simulink model "BraccioWithMotorsAndPIDandRL2020"  (R2020a)
settings: Solver=ode1be  StartTime=0.0  StopTime=14  FixedStep=0.01  RelTol=1e-3
values from neighbouring files (symbols this model uses):
  Z = [error; uold]    [RLNoLoop.m]
undefined symbols (not defined in the file or in its folder): X, Y
libraries: sm_lib x156, nesl_utility x52, simulink x12
(part 5 of 5)

== system BraccioWithMotorsAndPIDandRL2020/Subsystem3/link2 ==
  ReferenceFrame : sm_lib/Frames and Transforms/Reference Frame
  elbow_AxisTransform : sm_lib/Frames and Transforms/Rigid Transform  TranslationMethod=Cartesian  TranslationStandardOffset=0  TranslationStandardOffsetUnits=m  TranslationStandardAxis=+Z  TranslationCartesianOffset=[0, 0, 0]  TranslationCartesianOffsetUnits=m  TranslationROffset=0  TranslationROffsetUnits=m  TranslationZOffset=0  TranslationZOffsetUnits=m  TranslationThetaOffset=0  TranslationThetaOffsetUnits=deg  RotationMethod=ArbitraryAxis  RotationAngleUnits=rad  RotationStandardAxis=+Z  RotationAngle=1.570796326794897  RotationArbitraryAxis=[-0, 1, 0]  FollAlignAxisA=+X  BaseAlignAxisA=+Y  FollAlignAxisB=+Y  BaseAlignAxisB=+Z  RotationSequenceAxes=FollowerAxes  RotationSequence=XYX  RotationSequenceAngles=[0 0 0]  RotationSequenceAnglesUnits=deg  RotationMatrix=[1 0 0; 0 1 0; 0 0 1]  Quaternion=[1 0 0 0]
  elbow_OriginTransform : sm_lib/Frames and Transforms/Rigid Transform  TranslationMethod=Cartesian  TranslationStandardOffset=0  TranslationStandardOffsetUnits=m  TranslationStandardAxis=+Z  TranslationCartesianOffset=[0, 0, 0.1205]  TranslationCartesianOffsetUnits=m  TranslationROffset=0  TranslationROffsetUnits=m  TranslationZOffset=0  TranslationZOffsetUnits=m  TranslationThetaOffset=0  TranslationThetaOffsetUnits=deg  RotationMethod=RotationSequence  RotationAngleUnits=deg  RotationStandardAxis=+Z  RotationAngle=0.0  RotationArbitraryAxis=[0 0 1]  FollAlignAxisA=+X  BaseAlignAxisA=+Y  FollAlignAxisB=+Y  BaseAlignAxisB=+Z  RotationSequenceAxes=BaseAxes  RotationSequence=XYZ  RotationSequenceAngles=[-1.570796326794897, 0, 0]  RotationSequenceAnglesUnits=rad  RotationMatrix=[1 0 0; 0 1 0; 0 0 1]  Quaternion=[1 0 0 0]
  shoulder_AxisInvTransform : sm_lib/Frames and Transforms/Rigid Transform  TranslationMethod=Cartesian  TranslationStandardOffset=0  TranslationStandardOffsetUnits=m  TranslationStandardAxis=+Z  TranslationCartesianOffset=[0, 0, 0]  TranslationCartesianOffsetUnits=m  TranslationROffset=0  TranslationROffsetUnits=m  TranslationZOffset=0  TranslationZOffsetUnits=m  TranslationThetaOffset=0  TranslationThetaOffsetUnits=deg  RotationMethod=ArbitraryAxis  RotationAngleUnits=rad  RotationStandardAxis=+Z  RotationAngle=1.570796326794897  RotationArbitraryAxis=[-0, 1, 0]  FollAlignAxisA=+X  BaseAlignAxisA=+Y  FollAlignAxisB=+Y  BaseAlignAxisB=+Z  RotationSequenceAxes=FollowerAxes  RotationSequence=XYX  RotationSequenceAngles=[0 0 0]  RotationSequenceAnglesUnits=deg  RotationMatrix=[1 0 0; 0 1 0; 0 0 1]  Quaternion=[1 0 0 0]
  F : PMIOPort  Side=Left
  F1 : PMIOPort  Port=2  Side=Right
  connections:
  ReferenceFrame/RConn1 -- elbow_OriginTransform/LConn1 -- shoulder_AxisInvTransform/LConn1
  elbow_AxisTransform/RConn1 -- F1/RConn1
  elbow_AxisTransform/LConn1 -- elbow_OriginTransform/RConn1
  shoulder_AxisInvTransform/RConn1 -- F/RConn1

== system BraccioWithMotorsAndPIDandRL2020/Subsystem3/link3 ==
  ReferenceFrame : sm_lib/Frames and Transforms/Reference Frame
  elbow_AxisInvTransform : sm_lib/Frames and Transforms/Rigid Transform  TranslationMethod=Cartesian  TranslationStandardOffset=0  TranslationStandardOffsetUnits=m  TranslationStandardAxis=+Z  TranslationCartesianOffset=[0, 0, 0]  TranslationCartesianOffsetUnits=m  TranslationROffset=0  TranslationROffsetUnits=m  TranslationZOffset=0  TranslationZOffsetUnits=m  TranslationThetaOffset=0  TranslationThetaOffsetUnits=deg  RotationMethod=ArbitraryAxis  RotationAngleUnits=rad  RotationStandardAxis=+Z  RotationAngle=1.570796326794897  RotationArbitraryAxis=[-0, 1, 0]  FollAlignAxisA=+X  BaseAlignAxisA=+Y  FollAlignAxisB=+Y  BaseAlignAxisB=+Z  RotationSequenceAxes=FollowerAxes  RotationSequence=XYX  RotationSequenceAngles=[0 0 0]  RotationSequenceAnglesUnits=deg  RotationMatrix=[1 0 0; 0 1 0; 0 0 1]  Quaternion=[1 0 0 0]
  wrist_pitch_AxisTransform : sm_lib/Frames and Transforms/Rigid Transform  TranslationMethod=Cartesian  TranslationStandardOffset=0  TranslationStandardOffsetUnits=m  TranslationStandardAxis=+Z  TranslationCartesianOffset=[0, 0, 0]  TranslationCartesianOffsetUnits=m  TranslationROffset=0  TranslationROffsetUnits=m  TranslationZOffset=0  TranslationZOffsetUnits=m  TranslationThetaOffset=0  TranslationThetaOffsetUnits=deg  RotationMethod=ArbitraryAxis  RotationAngleUnits=rad  RotationStandardAxis=+Z  RotationAngle=1.570796326794897  RotationArbitraryAxis=[-0, 1, 0]  FollAlignAxisA=+X  BaseAlignAxisA=+Y  FollAlignAxisB=+Y  BaseAlignAxisB=+Z  RotationSequenceAxes=FollowerAxes  RotationSequence=XYX  RotationSequenceAngles=[0 0 0]  RotationSequenceAnglesUnits=deg  RotationMatrix=[1 0 0; 0 1 0; 0 0 1]  Quaternion=[1 0 0 0]
  wrist_pitch_OriginTransform : sm_lib/Frames and Transforms/Rigid Transform  TranslationMethod=Cartesian  TranslationStandardOffset=0  TranslationStandardOffsetUnits=m  TranslationStandardAxis=+Z  TranslationCartesianOffset=[0, 0, 0.1205]  TranslationCartesianOffsetUnits=m  TranslationROffset=0  TranslationROffsetUnits=m  TranslationZOffset=0  TranslationZOffsetUnits=m  TranslationThetaOffset=0  TranslationThetaOffsetUnits=deg  RotationMethod=RotationSequence  RotationAngleUnits=deg  RotationStandardAxis=+Z  RotationAngle=0.0  RotationArbitraryAxis=[0 0 1]  FollAlignAxisA=+X  BaseAlignAxisA=+Y  FollAlignAxisB=+Y  BaseAlignAxisB=+Z  RotationSequenceAxes=BaseAxes  RotationSequence=XYZ  RotationSequenceAngles=[-1.570796326794897, 0, 0]  RotationSequenceAnglesUnits=rad  RotationMatrix=[1 0 0; 0 1 0; 0 0 1]  Quaternion=[1 0 0 0]
  F : PMIOPort  Side=Left
  F1 : PMIOPort  Port=2  Side=Right
  connections:
  ReferenceFrame/RConn1 -- elbow_AxisInvTransform/LConn1 -- wrist_pitch_OriginTransform/LConn1
  elbow_AxisInvTransform/RConn1 -- F/RConn1
  wrist_pitch_AxisTransform/RConn1 -- F1/RConn1
  wrist_pitch_AxisTransform/LConn1 -- wrist_pitch_OriginTransform/RConn1

== system BraccioWithMotorsAndPIDandRL2020/Subsystem3/link4 ==
  ReferenceFrame : sm_lib/Frames and Transforms/Reference Frame
  wrist_pitch_AxisInvTransform : sm_lib/Frames and Transforms/Rigid Transform  TranslationMethod=Cartesian  TranslationStandardOffset=0  TranslationStandardOffsetUnits=m  TranslationStandardAxis=+Z  TranslationCartesianOffset=[0, 0, 0]  TranslationCartesianOffsetUnits=m  TranslationROffset=0  TranslationROffsetUnits=m  TranslationZOffset=0  TranslationZOffsetUnits=m  TranslationThetaOffset=0  TranslationThetaOffsetUnits=deg  RotationMethod=ArbitraryAxis  RotationAngleUnits=rad  RotationStandardAxis=+Z  RotationAngle=1.570796326794897  RotationArbitraryAxis=[-0, 1, 0]  FollAlignAxisA=+X  BaseAlignAxisA=+Y  FollAlignAxisB=+Y  BaseAlignAxisB=+Z  RotationSequenceAxes=FollowerAxes  RotationSequence=XYX  RotationSequenceAngles=[0 0 0]  RotationSequenceAnglesUnits=deg  RotationMatrix=[1 0 0; 0 1 0; 0 0 1]  Quaternion=[1 0 0 0]
  wrist_roll_AxisTransform : sm_lib/Frames and Transforms/Rigid Transform  TranslationMethod=Cartesian  TranslationStandardOffset=0  TranslationStandardOffsetUnits=m  TranslationStandardAxis=+Z  TranslationCartesianOffset=[0, 0, 0]  TranslationCartesianOffsetUnits=m  TranslationROffset=0  TranslationROffsetUnits=m  TranslationZOffset=0  TranslationZOffsetUnits=m  TranslationThetaOffset=0  TranslationThetaOffsetUnits=deg  RotationMethod=ArbitraryAxis  RotationAngleUnits=rad  RotationStandardAxis=+Z  RotationAngle=3.141592653589793  RotationArbitraryAxis=[1, 0, 0]  FollAlignAxisA=+X  BaseAlignAxisA=+Y  FollAlignAxisB=+Y  BaseAlignAxisB=+Z  RotationSequenceAxes=FollowerAxes  RotationSequence=XYX  RotationSequenceAngles=[0 0 0]  RotationSequenceAnglesUnits=deg  RotationMatrix=[1 0 0; 0 1 0; 0 0 1]  Quaternion=[1 0 0 0]
  wrist_roll_OriginTransform : sm_lib/Frames and Transforms/Rigid Transform  TranslationMethod=Cartesian  TranslationStandardOffset=0  TranslationStandardOffsetUnits=m  TranslationStandardAxis=+Z  TranslationCartesianOffset=[0, 0, 0.06]  TranslationCartesianOffsetUnits=m  TranslationROffset=0  TranslationROffsetUnits=m  TranslationZOffset=0  TranslationZOffsetUnits=m  TranslationThetaOffset=0  TranslationThetaOffsetUnits=deg  RotationMethod=RotationSequence  RotationAngleUnits=deg  RotationStandardAxis=+Z  RotationAngle=0.0  RotationArbitraryAxis=[0 0 1]  FollAlignAxisA=+X  BaseAlignAxisA=+Y  FollAlignAxisB=+Y  BaseAlignAxisB=+Z  RotationSequenceAxes=BaseAxes  RotationSequence=XYZ  RotationSequenceAngles=[0, 0, 0]  RotationSequenceAnglesUnits=rad  RotationMatrix=[1 0 0; 0 1 0; 0 0 1]  Quaternion=[1 0 0 0]
  F : PMIOPort  Side=Left
  F1 : PMIOPort  Port=2  Side=Right
  connections:
  ReferenceFrame/RConn1 -- wrist_pitch_AxisInvTransform/LConn1 -- wrist_roll_OriginTransform/LConn1
  wrist_pitch_AxisInvTransform/RConn1 -- F/RConn1
  wrist_roll_AxisTransform/RConn1 -- F1/RConn1
  wrist_roll_AxisTransform/LConn1 -- wrist_roll_OriginTransform/RConn1

== system BraccioWithMotorsAndPIDandRL2020/Subsystem3/link5 ==
  ReferenceFrame : sm_lib/Frames and Transforms/Reference Frame
  gripper_base_OriginTransform : sm_lib/Frames and Transforms/Rigid Transform  TranslationMethod=Cartesian  TranslationStandardOffset=0  TranslationStandardOffsetUnits=m  TranslationStandardAxis=+Z  TranslationCartesianOffset=[0, 0, 0.0065]  TranslationCartesianOffsetUnits=m  TranslationROffset=0  TranslationROffsetUnits=m  TranslationZOffset=0  TranslationZOffsetUnits=m  TranslationThetaOffset=0  TranslationThetaOffsetUnits=deg  RotationMethod=RotationSequence  RotationAngleUnits=deg  RotationStandardAxis=+Z  RotationAngle=0.0  RotationArbitraryAxis=[0 0 1]  FollAlignAxisA=+X  BaseAlignAxisA=+Y  FollAlignAxisB=+Y  BaseAlignAxisB=+Z  RotationSequenceAxes=BaseAxes  RotationSequence=XYZ  RotationSequenceAngles=[0, 0, 0]  RotationSequenceAnglesUnits=rad  RotationMatrix=[1 0 0; 0 1 0; 0 0 1]  Quaternion=[1 0 0 0]
  wrist_roll_AxisInvTransform : sm_lib/Frames and Transforms/Rigid Transform  TranslationMethod=Cartesian  TranslationStandardOffset=0  TranslationStandardOffsetUnits=m  TranslationStandardAxis=+Z  TranslationCartesianOffset=[0, 0, 0]  TranslationCartesianOffsetUnits=m  TranslationROffset=0  TranslationROffsetUnits=m  TranslationZOffset=0  TranslationZOffsetUnits=m  TranslationThetaOffset=0  TranslationThetaOffsetUnits=deg  RotationMethod=ArbitraryAxis  RotationAngleUnits=rad  RotationStandardAxis=+Z  RotationAngle=3.141592653589793  RotationArbitraryAxis=[1, 0, 0]  FollAlignAxisA=+X  BaseAlignAxisA=+Y  FollAlignAxisB=+Y  BaseAlignAxisB=+Z  RotationSequenceAxes=FollowerAxes  RotationSequence=XYX  RotationSequenceAngles=[0 0 0]  RotationSequenceAnglesUnits=deg  RotationMatrix=[1 0 0; 0 1 0; 0 0 1]  Quaternion=[1 0 0 0]
  F : PMIOPort  Side=Left
  F1 : PMIOPort  Port=2  Side=Right
  connections:
  ReferenceFrame/RConn1 -- gripper_base_OriginTransform/LConn1 -- wrist_roll_AxisInvTransform/LConn1
  gripper_base_OriginTransform/RConn1 -- F1/RConn1
  wrist_roll_AxisInvTransform/RConn1 -- F/RConn1

== matlab function BraccioWithMotorsAndPIDandRL2020/MATLAB Function ==
  data: u input; yd output
function yd = Desired_Trajectory(u)


yd = 1+0.5*cos((2*pi/20)*u+pi/10);

== matlab function BraccioWithMotorsAndPIDandRL2020/MATLAB Function2 ==
  settings: updateMethod=DISCRETE
  data: error input; u output
function u = NewRL (error)
%flag to the first run to put intial conditions
%allocates memory for it only once during the first call to the function
%use isempty in first use as it asiigned only place in memory
%without out any value so it is just empty place
persistent Flag
persistent Wa
persistent Wc
persistent Eold
persistent Eolder
persistent Uold
persistent wcuu
persistent wcue
persistent uPervious

%Intialize now all needed
%In if block to ensure it's set only once
if isempty(Flag)
    %Make the flag any value to leave the loop
    %by initializing a Persistent Variable
    Flag=5;

    %the old error will be set for the first time but later we get it
    Eold=0;
    Eolder=0;
    
    %First Wa make intial guess (2*2)
    P=0.073;
    wa1=P;
    wa2=-P;
    Wa=[wa1,wa2];

    %the old output response
    Uold=0;
    uPervious=0;

    %First Wc make initial guess (3*3)
    wcuu=1;
    wcue=-wcuu*Wa;
    Wc=[1,0,wcue(1);
        0,1,wcue(2);
        wcue(1),wcue(2),wcuu];  %(3*3)

    wcue=Wc(3,1:2);
    wcuu=Wc(3,3);

end

%Things to define again instead of persistent as it no updated
%assign values for alpha to be used later in Wa and Wc
%random value for R and i may make it something small like 0.01
% R = rand(1, 1); DOnt use random to have same performance
R=0.01;
Q=eye(2);
alphaC=0.000009;
alphaA=0.00000055;

%Things Change Every time
Eo=[Eold;Eolder];   %(2*1)
Er=[error;Eold];%(2*1)


r = 200;
while (r>0)           
    %Cost function
    cost=0.5*(Eo'*Q*Eo+Uold'*R*Uold); 
    Uest=-pinv(wcuu)*wcue*Er;
    Zk1=[error;Eold;Uest];
    Zold=[Eold;Eolder;Uold];

    %Qk approximate = 0.5 * Zk transpose * Wc * Zk
    %Zk is [Eold(1*1) ; u(1*1)]
    %Mu_K is the old output lets call it uold
    %Xk = [Old error (E_old); ]

    Qapp=0.5*Zold'*Wc*Zold;
    %Q next for k+1
    Qnext=0.5*Zk1'*Wc*Zk1;
    %Qdesire
    Qdes=cost+Qnext;

    %Wc (Tuning law)
    Wc=Wc-alphaC*(Qapp-Qdes)*(Zold*Zold');
    wcue=Wc(3,1:2);
    wcuu=Wc(3,3);

    %estimate the u_est
    Uapp=Wa*Eo;
    %u_desire
    Udes=-pinv(wcuu)*wcue*Eo;
    %Wa
    Wa=Wa-alphaA*(Uapp-Udes)*(Eo');
 
    %Calculate the new action u for the loop
    Uold=Wa*Er;

    if (abs(Uapp-Udes)>0.001)
        break;
    end

    r=r-1;
end 

%Assign the input error to Eold (error = desired - feedback) to be later
%used in next respond
Eolder=Eold;
Eold=error; 

%Calculate the new action u
Uold=Wa*Er;
u=uPervious+Uold;
uPervious=u;

== matlab function BraccioWithMotorsAndPIDandRL2020/MATLAB Function3 ==
  settings: updateMethod=DISCRETE
  data: error input; u output
function u = NewRL (error)
%flag to the first run to put intial conditions
%allocates memory for it only once during the first call to the function
%use isempty in first use as it asiigned only place in memory
%without out any value so it is just empty place
persistent Flag
persistent Wa
persistent Wc
persistent Eold
persistent Eolder
persistent Uold
persistent wcuu
persistent wcue
persistent uPervious

%Intialize now all needed
%In if block to ensure it's set only once
if isempty(Flag)
    %Make the flag any value to leave the loop
    %by initializing a Persistent Variable
    Flag=5;

    %the old error will be set for the first time but later we get it
    Eold=0;
    Eolder=0;
    
    %First Wa make intial guess (2*2)
    P=0.0316;
    wa1=P;
    wa2=-P;
    Wa=[wa1,wa2];

    %the old output response
    Uold=0;
    uPervious=0;

    %First Wc make initial guess (3*3)
    wcuu=1;
    wcue=-wcuu*Wa;
    Wc=[1,0,wcue(1);
        0,1,wcue(2);
        wcue(1),wcue(2),wcuu];  %(3*3)

    wcue=Wc(3,1:2);
    wcuu=Wc(3,3);

end

%Things to define again instead of persistent as it no updated
%assign values for alpha to be used later in Wa and Wc
%random value for R and i may make it something small like 0.01
% R = rand(1, 1); DOnt use random to have same performance
R=0.01;
Q=eye(2);
alphaC=0.000009;
alphaA=0.00000055;

%Things Change Every time
Eo=[Eold;Eolder];   %(2*1)
Er=[error;Eold];%(2*1)


r = 200;
while (r>0)           
    %Cost function
    cost=0.5*(Eo'*Q*Eo+Uold'*R*Uold); 
    Uest=-pinv(wcuu)*wcue*Er;
    Zk1=[error;Eold;Uest];
    Zold=[Eold;Eolder;Uold];

    %Qk approximate = 0.5 * Zk transpose * Wc * Zk
    %Zk is [Eold(1*1) ; u(1*1)]
    %Mu_K is the old output lets call it uold
    %Xk = [Old error (E_old); ]

    Qapp=0.5*Zold'*Wc*Zold;
    %Q next for k+1
    Qnext=0.5*Zk1'*Wc*Zk1;
    %Qdesire
    Qdes=cost+Qnext;

    %Wc (Tuning law)
    Wc=Wc-alphaC*(Qapp-Qdes)*(Zold*Zold');
    wcue=Wc(3,1:2);
    wcuu=Wc(3,3);

    %estimate the u_est
    Uapp=Wa*Eo;
    %u_desire
    Udes=-pinv(wcuu)*wcue*Eo;
    %Wa
    Wa=Wa-alphaA*(Uapp-Udes)*(Eo');
 
    %Calculate the new action u for the loop
    Uold=Wa*Er;

    if (abs(Uapp-Udes)>0.001)
        break;
    end

    r=r-1;
end 

%Assign the input error to Eold (error = desired - feedback) to be later
%used in next respond
Eolder=Eold;
Eold=error; 

%Calculate the new action u
Uold=Wa*Er;
u=uPervious+Uold;
uPervious=u;

== matlab function BraccioWithMotorsAndPIDandRL2020/MATLAB Function4 ==
  settings: updateMethod=DISCRETE
  data: error input; u output
function u = NewRL (error)
%flag to the first run to put intial conditions
%allocates memory for it only once during the first call to the function
%use isempty in first use as it asiigned only place in memory
%without out any value so it is just empty place
persistent Flag
persistent Wa
persistent Wc
persistent Eold
persistent Eolder
persistent Uold
persistent wcuu
persistent wcue
persistent uPervious

%Intialize now all needed
%In if block to ensure it's set only once
if isempty(Flag)
    %Make the flag any value to leave the loop
    %by initializing a Persistent Variable
    Flag=5;

    %the old error will be set for the first time but later we get it
    Eold=0;
    Eolder=0;
    
    %First Wa make intial guess (2*2)
    P=0.061;
    wa1=P;
    wa2=-P;
    Wa=[wa1,wa2];

    %the old output response
    Uold=0;
    uPervious=0;

    %First Wc make initial guess (3*3)
    wcuu=1;
    wcue=-wcuu*Wa;
    Wc=[1,0,wcue(1);
        0,1,wcue(2);
        wcue(1),wcue(2),wcuu];  %(3*3)

    wcue=Wc(3,1:2);
    wcuu=Wc(3,3);

end

%Things to define again instead of persistent as it no updated
%assign values for alpha to be used later in Wa and Wc
%random value for R and i may make it something small like 0.01
% R = rand(1, 1); DOnt use random to have same performance
R=0.01;
Q=eye(2);
alphaC=0.000009;
alphaA=0.00000055;

%Things Change Every time
Eo=[Eold;Eolder];   %(2*1)
Er=[error;Eold];%(2*1)


r = 200;
while (r>0)           
    %Cost function
    cost=0.5*(Eo'*Q*Eo+Uold'*R*Uold); 
    Uest=-pinv(wcuu)*wcue*Er;
    Zk1=[error;Eold;Uest];
    Zold=[Eold;Eolder;Uold];

    %Qk approximate = 0.5 * Zk transpose * Wc * Zk
    %Zk is [Eold(1*1) ; u(1*1)]
    %Mu_K is the old output lets call it uold
    %Xk = [Old error (E_old); ]

    Qapp=0.5*Zold'*Wc*Zold;
    %Q next for k+1
    Qnext=0.5*Zk1'*Wc*Zk1;
    %Qdesire
    Qdes=cost+Qnext;

    %Wc (Tuning law)
    Wc=Wc-alphaC*(Qapp-Qdes)*(Zold*Zold');
    wcue=Wc(3,1:2);
    wcuu=Wc(3,3);

    %estimate the u_est
    Uapp=Wa*Eo;
    %u_desire
    Udes=-pinv(wcuu)*wcue*Eo;
    %Wa
    Wa=Wa-alphaA*(Uapp-Udes)*(Eo');
 
    %Calculate the new action u for the loop
    Uold=Wa*Er;

    if (abs(Uapp-Udes)>0.001)
        break;
    end

    r=r-1;
end 

%Assign the input error to Eold (error = desired - feedback) to be later
%used in next respond
Eolder=Eold;
Eold=error; 

%Calculate the new action u
Uold=Wa*Er;
u=uPervious+Uold;
uPervious=u;

== matlab function BraccioWithMotorsAndPIDandRL2020/MATLAB Function5 ==
  settings: updateMethod=DISCRETE
  data: error input; u output
function u = NewRL (error)
%flag to the first run to put intial conditions
%allocates memory for it only once during the first call to the function
%use isempty in first use as it asiigned only place in memory
%without out any value so it is just empty place
persistent Flag
persistent Wa
persistent Wc
persistent Eold
persistent Eolder
persistent Uold
persistent wcuu
persistent wcue
persistent uPervious

%Intialize now all needed
%In if block to ensure it's set only once
if isempty(Flag)
    %Make the flag any value to leave the loop
    %by initializing a Persistent Variable
    Flag=5;

    %the old error will be set for the first time but later we get it
    Eold=0;
    Eolder=0;
    
    %First Wa make intial guess (2*2)
    P=0.0558;
    wa1=P;
    wa2=-P;
    Wa=[wa1,wa2];

    %the old output response
    Uold=0;
    uPervious=0;

    %First Wc make initial guess (3*3)
    wcuu=1;
    wcue=-wcuu*Wa;
    Wc=[1,0,wcue(1);
        0,1,wcue(2);
        wcue(1),wcue(2),wcuu];  %(3*3)

    wcue=Wc(3,1:2);
    wcuu=Wc(3,3);

end

%Things to define again instead of persistent as it no updated
%assign values for alpha to be used later in Wa and Wc
%random value for R and i may make it something small like 0.01
% R = rand(1, 1); DOnt use random to have same performance
R=0.01;
Q=eye(2);
alphaC=0.000009;
alphaA=0.00000055;

%Things Change Every time
Eo=[Eold;Eolder];   %(2*1)
Er=[error;Eold];%(2*1)


r = 200;
while (r>0)           
    %Cost function
    cost=0.5*(Eo'*Q*Eo+Uold'*R*Uold); 
    Uest=-pinv(wcuu)*wcue*Er;
    Zk1=[error;Eold;Uest];
    Zold=[Eold;Eolder;Uold];

    %Qk approximate = 0.5 * Zk transpose * Wc * Zk
    %Zk is [Eold(1*1) ; u(1*1)]
    %Mu_K is the old output lets call it uold
    %Xk = [Old error (E_old); ]

    Qapp=0.5*Zold'*Wc*Zold;
    %Q next for k+1
    Qnext=0.5*Zk1'*Wc*Zk1;
    %Qdesire
    Qdes=cost+Qnext;

    %Wc (Tuning law)
    Wc=Wc-alphaC*(Qapp-Qdes)*(Zold*Zold');
    wcue=Wc(3,1:2);
    wcuu=Wc(3,3);

    %estimate the u_est
    Uapp=Wa*Eo;
    %u_desire
    Udes=-pinv(wcuu)*wcue*Eo;
    %Wa
    Wa=Wa-alphaA*(Uapp-Udes)*(Eo');
 
    %Calculate the new action u for the loop
    Uold=Wa*Er;

    if (abs(Uapp-Udes)>0.001)
        break;
    end

    r=r-1;
end 

%Assign the input error to Eold (error = desired - feedback) to be later
%used in next respond
Eolder=Eold;
Eold=error; 

%Calculate the new action u
Uold=Wa*Er;
u=uPervious+Uold;
uPervious=u;

== matlab function BraccioWithMotorsAndPIDandRL2020/MATLAB Function6 ==
  settings: updateMethod=DISCRETE
  data: error input; u output
function u = RL_1 (error)
%flag to the first run to put intial conditions
%allocates memory for it only once during the first call to the function
%use isempty in first use as it asiigned only place in memory
%without out any value so it is just empty place
persistent flag
persistent Wc
persistent Wa
persistent Eold
persistent uold

%Intialize now all needed
%In if block to ensure it's set only once
if isempty(flag)
    %First Wa make intial guess (1*1)
    P=0.04372;

    Wa= P;
    
    %First Wc make initial guess (2*2)
    Wc=[1,     -P;
        -P,  1];
    
    %the old output response
    uold = 0;

    %the old error will be set for the first time but later we get it
    Eold = 0;

    %Make the flag any value to leave the loop
    %by initializing a Persistent Variable
    flag = 5;
end
%Things to define again instead of persistent as it no updated
    %assign values for alpha to be used later in Wa and Wc
    alpha_A=0.006;
    alpha_C=0.0004;
    %Let the Q to be 0.7
    Q=0.4;

    %random value for R and i may make it something small like 0.01
    % R = rand(1, 1); DOnt use random to have same performance
    R = 0.08;

%Things Change Every time
Z = [error; uold];
Zold = [Eold; uold];

%RL
%Q next for k+1
Qnext = 0.5 * Z' * Wc * Z;

%Cost function
Cost = Eold' * Q * Eold + uold' * R * uold;

%Qdesire
Qdesire = Cost + Qnext;

%Qk approximate = 0.5 * Zk transpose * Wc * Zk
%Zk is [Eold(1*1) ; u(1*1)]
%Mu_K is the old output lets call it uold
%Xk = [Old error (E_old); ]
Qapp = 0.5 * Zold' * Wc * Zold;

%Wc (Tuning law)
Wc = Wc - alpha_C * (Qapp - Qdesire) * (Zold*Zold');

%
Wcu = -Wc(2,2) * Wa;

%u_desire
u_desire = - inv(Wc(2,2)) * Wcu * error;

%estimate the u_est
%(1*1) * (1*1)
u_est = Wa * error;

%Wa
Wa = Wa - alpha_A * (u_est - u_desire) * (Eold');

%Calculate the new action u
u = uold + Wa * error;

%Assign the input error to Eold (error = desired - feedback) to be later
%used in next respond
Eold = error;

end

== matlab function BraccioWithMotorsAndPIDandRL2020/MATLAB Function10 ==
  settings: updateMethod=DISCRETE
  data: error input; u output
function u = NewRL (error)
%flag to the first run to put intial conditions
%allocates memory for it only once during the first call to the function
%use isempty in first use as it asiigned only place in memory
%without out any value so it is just empty place
persistent Flag
persistent Wa
persistent Wc
persistent Eold
persistent Eolder
persistent Uold
persistent wcuu
persistent wcue
persistent uPervious

%Intialize now all needed
%In if block to ensure it's set only once
if isempty(Flag)
    %Make the flag any value to leave the loop
    %by initializing a Persistent Variable
    Flag=5;

    %the old error will be set for the first time but later we get it
    Eold=0;
    Eolder=0;
    
    %First Wa make intial guess (2*2)
    P=0.061;
    wa1=P;
    wa2=-P;
    Wa=[wa1,wa2];

    %the old output response
    Uold=0;
    uPervious=0;

    %First Wc make initial guess (3*3)
    wcuu=1;
    wcue=-wcuu*Wa;
    Wc=[1,0,wcue(1);
        0,1,wcue(2);
        wcue(1),wcue(2),wcuu];  %(3*3)

    wcue=Wc(3,1:2);
    wcuu=Wc(3,3);

end

%Things to define again instead of persistent as it no updated
%assign values for alpha to be used later in Wa and Wc
%random value for R and i may make it something small like 0.01
% R = rand(1, 1); DOnt use random to have same performance
R=0.01;
Q=eye(2);
alphaC=0.000009;
alphaA=0.00000055;

%Things Change Every time
Eo=[Eold;Eolder];   %(2*1)
Er=[error;Eold];%(2*1)


r = 200;
while (r>0)           
    %Cost function
    cost=0.5*(Eo'*Q*Eo+Uold'*R*Uold); 
    Uest=-pinv(wcuu)*wcue*Er;
    Zk1=[error;Eold;Uest];
    Zold=[Eold;Eolder;Uold];

    %Qk approximate = 0.5 * Zk transpose * Wc * Zk
    %Zk is [Eold(1*1) ; u(1*1)]
    %Mu_K is the old output lets call it uold
    %Xk = [Old error (E_old); ]

    Qapp=0.5*Zold'*Wc*Zold;
    %Q next for k+1
    Qnext=0.5*Zk1'*Wc*Zk1;
    %Qdesire
    Qdes=cost+Qnext;

    %Wc (Tuning law)
    Wc=Wc-alphaC*(Qapp-Qdes)*(Zold*Zold');
    wcue=Wc(3,1:2);
    wcuu=Wc(3,3);

    %estimate the u_est
    Uapp=Wa*Eo;
    %u_desire
    Udes=-pinv(wcuu)*wcue*Eo;
    %Wa
    Wa=Wa-alphaA*(Uapp-Udes)*(Eo');
 
    %Calculate the new action u for the loop
    Uold=Wa*Er;

    if (abs(Uapp-Udes)>0.001)
        break;
    end

    r=r-1;
end 

%Assign the input error to Eold (error = desired - feedback) to be later
%used in next respond
Eolder=Eold;
Eold=error; 

%Calculate the new action u
Uold=Wa*Er;
u=uPervious+Uold;
uPervious=u;

== matlab function BraccioWithMotorsAndPIDandRL2020/MATLAB Function11 ==
  settings: updateMethod=DISCRETE
  data: error input; u output
function u = NewRL (error)
%flag to the first run to put intial conditions
%allocates memory for it only once during the first call to the function
%use isempty in first use as it asiigned only place in memory
%without out any value so it is just empty place
persistent Flag
persistent Wa
persistent Wc
persistent Eold
persistent Eolder
persistent Uold
persistent wcuu
persistent wcue
persistent uPervious

%Intialize now all needed
%In if block to ensure it's set only once
if isempty(Flag)
    %Make the flag any value to leave the loop
    %by initializing a Persistent Variable
    Flag=5;

    %the old error will be set for the first time but later we get it
    Eold=0;
    Eolder=0;
    
    %First Wa make intial guess (2*2)
    P=0.0558;
    wa1=P;
    wa2=-P;
    Wa=[wa1,wa2];

    %the old output response
    Uold=0;
    uPervious=0;

    %First Wc make initial guess (3*3)
    wcuu=1;
    wcue=-wcuu*Wa;
    Wc=[1,0,wcue(1);
        0,1,wcue(2);
        wcue(1),wcue(2),wcuu];  %(3*3)

    wcue=Wc(3,1:2);
    wcuu=Wc(3,3);

end

%Things to define again instead of persistent as it no updated
%assign values for alpha to be used later in Wa and Wc
%random value for R and i may make it something small like 0.01
% R = rand(1, 1); DOnt use random to have same performance
R=0.01;
Q=eye(2);
alphaC=0.000009;
alphaA=0.00000055;

%Things Change Every time
Eo=[Eold;Eolder];   %(2*1)
Er=[error;Eold];%(2*1)


r = 200;
while (r>0)           
    %Cost function
    cost=0.5*(Eo'*Q*Eo+Uold'*R*Uold); 
    Uest=-pinv(wcuu)*wcue*Er;
    Zk1=[error;Eold;Uest];
    Zold=[Eold;Eolder;Uold];

    %Qk approximate = 0.5 * Zk transpose * Wc * Zk
    %Zk is [Eold(1*1) ; u(1*1)]
    %Mu_K is the old output lets call it uold
    %Xk = [Old error (E_old); ]

    Qapp=0.5*Zold'*Wc*Zold;
    %Q next for k+1
    Qnext=0.5*Zk1'*Wc*Zk1;
    %Qdesire
    Qdes=cost+Qnext;

    %Wc (Tuning law)
    Wc=Wc-alphaC*(Qapp-Qdes)*(Zold*Zold');
    wcue=Wc(3,1:2);
    wcuu=Wc(3,3);

    %estimate the u_est
    Uapp=Wa*Eo;
    %u_desire
    Udes=-pinv(wcuu)*wcue*Eo;
    %Wa
    Wa=Wa-alphaA*(Uapp-Udes)*(Eo');
 
    %Calculate the new action u for the loop
    Uold=Wa*Er;

    if (abs(Uapp-Udes)>0.001)
        break;
    end

    r=r-1;
end 

%Assign the input error to Eold (error = desired - feedback) to be later
%used in next respond
Eolder=Eold;
Eold=error; 

%Calculate the new action u
Uold=Wa*Er;
u=uPervious+Uold;
uPervious=u;

== matlab function BraccioWithMotorsAndPIDandRL2020/MATLAB Function12 ==
  settings: updateMethod=DISCRETE
  data: error input; u output
function u = RL_1 (error)
%flag to the first run to put intial conditions
%allocates memory for it only once during the first call to the function
%use isempty in first use as it asiigned only place in memory
%without out any value so it is just empty place
persistent flag
persistent Wc
persistent Wa
persistent Eold
persistent uold

%Intialize now all needed
%In if block to ensure it's set only once
if isempty(flag)
    %First Wa make intial guess (1*1)
    P=0.04372;

    Wa= P;
    
    %First Wc make initial guess (2*2)
    Wc=[1,     -P;
        -P,  1];
    
    %the old output response
    uold = 0;

    %the old error will be set for the first time but later we get it
    Eold = 0;

    %Make the flag any value to leave the loop
    %by initializing a Persistent Variable
    flag = 5;
end
%Things to define again instead of persistent as it no updated
    %assign values for alpha to be used later in Wa and Wc
    alpha_A=0.006;
    alpha_C=0.0004;
    %Let the Q to be 0.7
    Q=0.4;

    %random value for R and i may make it something small like 0.01
    % R = rand(1, 1); DOnt use random to have same performance
    R = 0.08;

%Things Change Every time
Z = [error; uold];
Zold = [Eold; uold];

%RL
%Q next for k+1
Qnext = 0.5 * Z' * Wc * Z;

%Cost function
Cost = Eold' * Q * Eold + uold' * R * uold;

%Qdesire
Qdesire = Cost + Qnext;

%Qk approximate = 0.5 * Zk transpose * Wc * Zk
%Zk is [Eold(1*1) ; u(1*1)]
%Mu_K is the old output lets call it uold
%Xk = [Old error (E_old); ]
Qapp = 0.5 * Zold' * Wc * Zold;

%Wc (Tuning law)
Wc = Wc - alpha_C * (Qapp - Qdesire) * (Zold*Zold');

%
Wcu = -Wc(2,2) * Wa;

%u_desire
u_desire = - inv(Wc(2,2)) * Wcu * error;

%estimate the u_est
%(1*1) * (1*1)
u_est = Wa * error;

%Wa
Wa = Wa - alpha_A * (u_est - u_desire) * (Eold');

%Calculate the new action u
u = uold + Wa * error;

%Assign the input error to Eold (error = desired - feedback) to be later
%used in next respond
Eold = error;

end

== matlab function BraccioWithMotorsAndPIDandRL2020/MATLAB Function7 ==
  settings: updateMethod=DISCRETE
  data: error input; u output
function u = RL_1 (error)
%flag to the first run to put intial conditions
%allocates memory for it only once during the first call to the function
%use isempty in first use as it asiigned only place in memory
%without out any value so it is just empty place
persistent flag
persistent Wc
persistent Wa
persistent Eold
persistent uold

%Intialize now all needed
%In if block to ensure it's set only once
if isempty(flag)
    %First Wa make intial guess (1*1)
    P=0.026;

    Wa= P;
    
    %First Wc make initial guess (2*2)
    Wc=[1,     -P;
        -P,  1];
    
    %the old output response
    uold = 0;

    %the old error will be set for the first time but later we get it
    Eold = 0;

    %Make the flag any value to leave the loop
    %by initializing a Persistent Variable
    flag = 5;
end
%Things to define again instead of persistent as it no updated
    %assign values for alpha to be used later in Wa and Wc
    alpha_A=0.006;
    alpha_C=0.0004;
    %Let the Q to be 0.7
    Q=0.4;

    %random value for R and i may make it something small like 0.01
    % R = rand(1, 1); DOnt use random to have same performance
    R = 0.08;

%Things Change Every time
Z = [error; uold];
Zold = [Eold; uold];

%RL
%Q next for k+1
Qnext = 0.5 * Z' * Wc * Z;

%Cost function
Cost = Eold' * Q * Eold + uold' * R * uold;

%Qdesire
Qdesire = Cost + Qnext;

%Qk approximate = 0.5 * Zk transpose * Wc * Zk
%Zk is [Eold(1*1) ; u(1*1)]
%Mu_K is the old output lets call it uold
%Xk = [Old error (E_old); ]
Qapp = 0.5 * Zold' * Wc * Zold;

%Wc (Tuning law)
Wc = Wc - alpha_C * (Qapp - Qdesire) * (Zold*Zold');

%
Wcu = -Wc(2,2) * Wa;

%u_desire
u_desire = - inv(Wc(2,2)) * Wcu * error;

%estimate the u_est
%(1*1) * (1*1)
u_est = Wa * error;

%Wa
Wa = Wa - alpha_A * (u_est - u_desire) * (Eold');

%Calculate the new action u
u = uold + Wa * error;

%Assign the input error to Eold (error = desired - feedback) to be later
%used in next respond
Eold = error;

end

== matlab function BraccioWithMotorsAndPIDandRL2020/MATLAB Function1 ==
  settings: updateMethod=DISCRETE
  data: error input; u output
function u = RL_1 (error)
%flag to the first run to put intial conditions
%allocates memory for it only once during the first call to the function
%use isempty in first use as it asiigned only place in memory
%without out any value so it is just empty place
persistent flag
persistent Wc
persistent Wa
persistent Eold
persistent uold

%Intialize now all needed
%In if block to ensure it's set only once
if isempty(flag)
    %First Wa make intial guess (1*1)
    P=0.026;

    Wa= P;
    
    %First Wc make initial guess (2*2)
    Wc=[1,     -P;
        -P,  1];
    
    %the old output response
    uold = 0;

    %the old error will be set for the first time but later we get it
    Eold = 0;

    %Make the flag any value to leave the loop
    %by initializing a Persistent Variable
    flag = 5;
end
%Things to define again instead of persistent as it no updated
    %assign values for alpha to be used later in Wa and Wc
    alpha_A=0.006;
    alpha_C=0.0004;
    %Let the Q to be 0.4
    Q=0.4;

    %random value for R and i may make it something small like 0.01
    % R = rand(1, 1); DOnt use random to have same performance
    R = 0.08;

%Things Change Every time
Z = [error; uold];
Zold = [Eold; uold];

%RL
%Q next for k+1
Qnext = 0.5 * Z' * Wc * Z;

%Cost function
Cost = Eold' * Q * Eold + uold' * R * uold;

%Qdesire
Qdesire = Cost + Qnext;

%Qk approximate = 0.5 * Zk transpose * Wc * Zk
%Zk is [Eold(1*1) ; u(1*1)]
%Mu_K is the old output lets call it uold
%Xk = [Old error (E_old); ]
Qapp = 0.5 * Zold' * Wc * Zold;

%Wc (Tuning law)
Wc = Wc - alpha_C * (Qapp - Qdesire) * (Zold*Zold');

%
Wcu = -Wc(2,2) * Wa;

%u_desire
u_desire = - inv(Wc(2,2)) * Wcu * error;

%estimate the u_est
%(1*1) * (1*1)
u_est = Wa * error;

%Wa
Wa = Wa - alpha_A * (u_est - u_desire) * (Eold');

%Calculate the new action u
u = uold + Wa * error;

%Assign the input error to Eold (error = desired - feedback) to be later
%used in next respond
Eold = error;

end

== matlab function BraccioWithMotorsAndPIDandRL2020/MATLAB Function8 ==
  settings: updateMethod=DISCRETE
  data: error input; u output
function u = NewRL (error)
%flag to the first run to put intial conditions
%allocates memory for it only once during the first call to the function
%use isempty in first use as it asiigned only place in memory
%without out any value so it is just empty place
persistent Flag
persistent Wa
persistent Wc
persistent Eold
persistent Eolder
persistent Uold
persistent wcuu
persistent wcue
persistent uPervious

%Intialize now all needed
%In if block to ensure it's set only once
if isempty(Flag)
    %Make the flag any value to leave the loop
    %by initializing a Persistent Variable
    Flag=5;

    %the old error will be set for the first time but later we get it
    Eold=0;
    Eolder=0;
    
    %First Wa make intial guess (2*2)
    P=0.073;
    wa1=P;
    wa2=-P;
    Wa=[wa1,wa2];

    %the old output response
    Uold=0;
    uPervious=0;

    %First Wc make initial guess (3*3)
    wcuu=1;
    wcue=-wcuu*Wa;
    Wc=[1,0,wcue(1);
        0,1,wcue(2);
        wcue(1),wcue(2),wcuu];  %(3*3)

    wcue=Wc(3,1:2);
    wcuu=Wc(3,3);

end

%Things to define again instead of persistent as it no updated
%assign values for alpha to be used later in Wa and Wc
%random value for R and i may make it something small like 0.01
% R = rand(1, 1); DOnt use random to have same performance
R=0.01;
Q=eye(2);
alphaC=0.000009;
alphaA=0.00000055;

%Things Change Every time
Eo=[Eold;Eolder];   %(2*1)
Er=[error;Eold];%(2*1)


r = 200;
while (r>0)           
    %Cost function
    cost=0.5*(Eo'*Q*Eo+Uold'*R*Uold); 
    Uest=-pinv(wcuu)*wcue*Er;
    Zk1=[error;Eold;Uest];
    Zold=[Eold;Eolder;Uold];

    %Qk approximate = 0.5 * Zk transpose * Wc * Zk
    %Zk is [Eold(1*1) ; u(1*1)]
    %Mu_K is the old output lets call it uold
    %Xk = [Old error (E_old); ]

    Qapp=0.5*Zold'*Wc*Zold;
    %Q next for k+1
    Qnext=0.5*Zk1'*Wc*Zk1;
    %Qdesire
    Qdes=cost+Qnext;

    %Wc (Tuning law)
    Wc=Wc-alphaC*(Qapp-Qdes)*(Zold*Zold');
    wcue=Wc(3,1:2);
    wcuu=Wc(3,3);

    %estimate the u_est
    Uapp=Wa*Eo;
    %u_desire
    Udes=-pinv(wcuu)*wcue*Eo;
    %Wa
    Wa=Wa-alphaA*(Uapp-Udes)*(Eo');
 
    %Calculate the new action u for the loop
    Uold=Wa*Er;

    if (abs(Uapp-Udes)>0.001)
        break;
    end

    r=r-1;
end 

%Assign the input error to Eold (error = desired - feedback) to be later
%used in next respond
Eolder=Eold;
Eold=error; 

%Calculate the new action u
Uold=Wa*Er;
u=uPervious+Uold;
uPervious=u;

== matlab function BraccioWithMotorsAndPIDandRL2020/MATLAB Function9 ==
  settings: updateMethod=DISCRETE
  data: error input; u output
function u = NewRL (error)
%flag to the first run to put intial conditions
%allocates memory for it only once during the first call to the function
%use isempty in first use as it asiigned only place in memory
%without out any value so it is just empty place
persistent Flag
persistent Wa
persistent Wc
persistent Eold
persistent Eolder
persistent Uold
persistent wcuu
persistent wcue
persistent uPervious

%Intialize now all needed
%In if block to ensure it's set only once
if isempty(Flag)
    %Make the flag any value to leave the loop
    %by initializing a Persistent Variable
    Flag=5;

    %the old error will be set for the first time but later we get it
    Eold=0;
    Eolder=0;
    
    %First Wa make intial guess (2*2)
    P=0.0316;
    wa1=P;
    wa2=-P;
    Wa=[wa1,wa2];

    %the old output response
    Uold=0;
    uPervious=0;

    %First Wc make initial guess (3*3)
    wcuu=1;
    wcue=-wcuu*Wa;
    Wc=[1,0,wcue(1);
        0,1,wcue(2);
        wcue(1),wcue(2),wcuu];  %(3*3)

    wcue=Wc(3,1:2);
    wcuu=Wc(3,3);

end

%Things to define again instead of persistent as it no updated
%assign values for alpha to be used later in Wa and Wc
%random value for R and i may make it something small like 0.01
% R = rand(1, 1); DOnt use random to have same performance
R=0.01;
Q=eye(2);
alphaC=0.000009;
alphaA=0.00000055;

%Things Change Every time
Eo=[Eold;Eolder];   %(2*1)
Er=[error;Eold];%(2*1)


r = 200;
while (r>0)           
    %Cost function
    cost=0.5*(Eo'*Q*Eo+Uold'*R*Uold); 
    Uest=-pinv(wcuu)*wcue*Er;
    Zk1=[error;Eold;Uest];
    Zold=[Eold;Eolder;Uold];

    %Qk approximate = 0.5 * Zk transpose * Wc * Zk
    %Zk is [Eold(1*1) ; u(1*1)]
    %Mu_K is the old output lets call it uold
    %Xk = [Old error (E_old); ]

    Qapp=0.5*Zold'*Wc*Zold;
    %Q next for k+1
    Qnext=0.5*Zk1'*Wc*Zk1;
    %Qdesire
    Qdes=cost+Qnext;

    %Wc (Tuning law)
    Wc=Wc-alphaC*(Qapp-Qdes)*(Zold*Zold');
    wcue=Wc(3,1:2);
    wcuu=Wc(3,3);

    %estimate the u_est
    Uapp=Wa*Eo;
    %u_desire
    Udes=-pinv(wcuu)*wcue*Eo;
    %Wa
    Wa=Wa-alphaA*(Uapp-Udes)*(Eo');
 
    %Calculate the new action u for the loop
    Uold=Wa*Er;

    if (abs(Uapp-Udes)>0.001)
        break;
    end

    r=r-1;
end 

%Assign the input error to Eold (error = desired - feedback) to be later
%used in next respond
Eolder=Eold;
Eold=error; 

%Calculate the new action u
Uold=Wa*Er;
u=uPervious+Uold;
uPervious=u;
